simulink model "MuscleEnergyTestModel"  (R2019b)
settings: Solver=ode15s  StartTime=0.0  StopTime=0.005  MaxStep=0.01  RelTol=1e-4  AbsTol=1e-6
values from neighbouring files (symbols this model uses):
  Ahill = 0.25    [MuscleEnergyTest.m]
  c = 0.05    [BodyMechParams.m]
  eref = 0.04    [BodyMechParams.m]
  Fmax = 4000    [MuscleEnergyTest.m]
  FT = 20    [MuscleEnergyTest.m]
  gmax = 1.5    [MuscleEnergyTest.m]
  K = 5    [BodyMechParams.m]
  lopt = 0.055    [MuscleEnergyTest.m]
  lslack = 0.245    [MuscleEnergyTest.m]
  N = 1.5    [BodyMechParams.m]    (also in cmaes.m = size(x,1); mergeCompareEnergyCosts.m = {S.name})
  stim_val = stimulations_val(i)    [MuscleEnergyTest.m]
  v_set = v_simulations(j)    [MuscleEnergyTest.m]
  vmax = 12    [MuscleEnergyTest.m]
  w = 0.56    [BodyMechParams.m]    (also in MuscleEnergyTest.m = 1.039; cmaes.m = ones(size(x,1)))
undefined symbols (not defined in the file or in its folder): iso_short_length
libraries: simulink x1, NeuroMuscularLibrary x1
settings Model: Creator=Nathan  LastModifiedBy=Nathan
settings DataIOCC: SaveFinalState=on  SaveFormat=StructureWithTime  SaveOutput=off  SaveState=on  ReturnWorkspaceOutputs=off

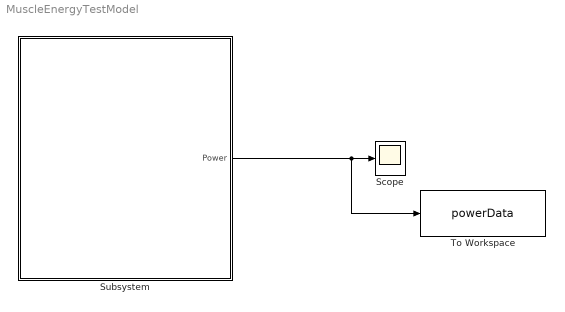
== system MuscleEnergyTestModel ==
  Scope : Scope
  Subsystem : Subsystem  mask{Fmax=Fmax, lopt=lopt, vmax=vmax, lslack=lslack, FT=FT, stim=stim_val, v_set=v_set}
      mask prompts: Fmax "Max Isometric Force in N"; lopt "Optimal Length in m"; vmax "Max Contraction Velocity in m/s"; lslack "Slack Length [m]"; FT "Percent Fast Twitch"; stim "Stimulation value"; v_set "Muscle velocity"
  To Workspace : ToWorkspace  VariableName=powerData  SampleTime=-1
  wires:
  Subsystem/1(Power) -> Scope/1, To Workspace/1

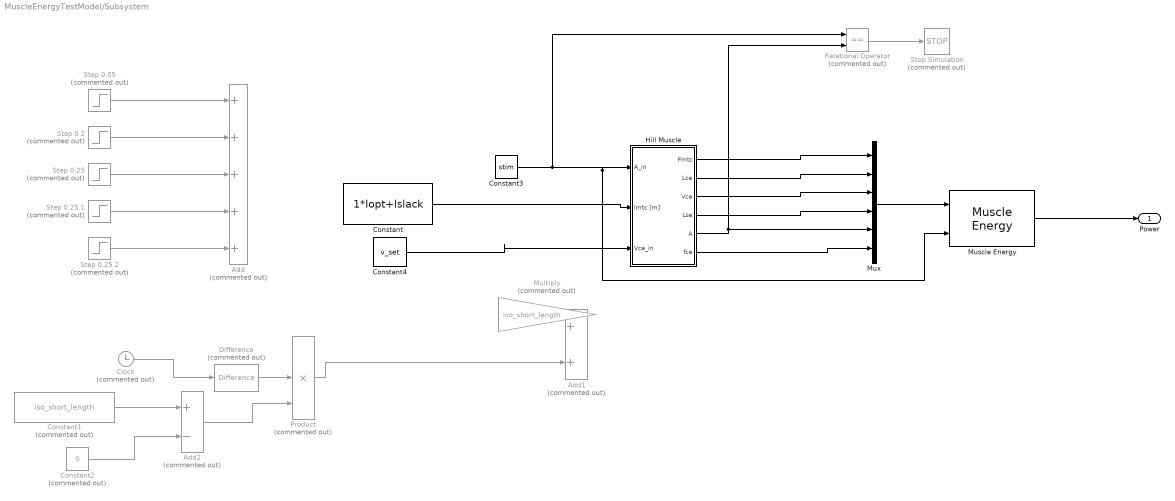
== system MuscleEnergyTestModel/Subsystem ==
  Add : Sum  Commented=on  Inputs=+++++
  Add1 : Sum  Commented=on
  Add2 : Sum  Commented=on  Inputs=+-
  Clock : Clock  Commented=on
      settings: Decimation=10000
  Constant : Constant  Value=1*lopt+lslack
  Constant1 : Constant  Commented=on  Value=iso_short_length
  Constant2 : Constant  Commented=on  Value=0
  Constant3 : Constant  Value=stim
  Constant4 : Constant  Value=v_set
  Difference : simulink/Discrete/Difference  Commented=on  ICPrevInput=0.0  OutMin=[]  OutMax=[]  OutDataType=fixdt(1, 16)  OutScaling=2^-10  DoSatur=off
  Hill Muscle : Subsystem  mask(Hill Type Muscle){Fmax=Fmax, lopt=lopt, vmax=vmax, lslack=lslack}
      mask prompts: Fmax "Max Isometric Force [N]"; lopt "Optimal Length [m]"; vmax "Max Contraction Velocity [m/s]"; lslack "Slack Length [m]"
      mask help:
      | Hill Type Muscle Model. This dialog allows you to specify several muscle-specific parameters. The block also requires several parameters to be defined globally in the matlab workspace:
      |
      | Excitation-contraction coupling parameters:
      | preA: preactivation
      | tau:  delay time constant [s]
      |
      | Contractile element (CE) force-length relationship:
      | w: width [lopt]
      | c: remaining force at +/- width
      |
      | CE force-velocity parameters:
      | N: eccentric force enhancement [Fmax]
      | K: shape factor
      |
      | Series elastic element (SE) force-length relationship
      | eref: tendon reference strain [lslack]
  Multiply : Gain  Commented=on  Gain=iso_short_length
  Muscle Energy : NeuroMuscularLibrary/Muscle Energy  lopt=lopt  FT=FT  Fmax=Fmax  vmax=vmax
  Mux : Mux  Inputs=6
  Product : Product  Commented=on  Inputs=3
  Relational Operator : RelationalOperator  Commented=on  Operator===  OutDataTypeStr=boolean  RndMeth=Simplest
  Step 0.05 : Step  Commented=on  After=0.05  SampleTime=0
  Step 0.2 : Step  Commented=on  Time=4  After=0.2  SampleTime=0
  Step 0.25 : Step  Commented=on  Time=7  After=0.25  SampleTime=0
  Step 0.25 1 : Step  Commented=on  Time=10  After=0.25  SampleTime=0
  Step 0.25 2 : Step  Commented=on  Time=13  After=0.25  SampleTime=0
  Stop Simulation : Stop  Commented=on
  Power : Outport
  wires:
  Mux/1 -> Muscle Energy/1
  Constant3/1 -> Relational Operator/1, Hill Muscle/1(A_in), Muscle Energy/2
  Hill Muscle/3(Vce) -> Mux/3
  Hill Muscle/4(Lse) -> Mux/4
  Hill Muscle/6(fce) -> Mux/6
  Hill Muscle/2(Lce) -> Mux/2
  Hill Muscle/1(Fmtc) -> Mux/1
  Constant/1 -> Hill Muscle/2(lmtc [m])
  Clock/1 -> Difference/1
  Difference/1 -> Product/2
  Product/1 -> Add1/2
  Add2/1 -> Product/3
  Constant1/1 -> Add2/1
  Constant2/1 -> Add2/2
  Muscle Energy/1 -> Power/1
  Step 0.05/1 -> Add/1
  Step 0.25 2/1 -> Add/5
  Step 0.25/1 -> Add/3
  Step 0.25 1/1 -> Add/4
  Step 0.2/1 -> Add/2
  Constant4/1 -> Hill Muscle/3(Vce_in)
  Relational Operator/1 -> Stop Simulation/1
  Hill Muscle/5(A) -> Relational Operator/2, Mux/5

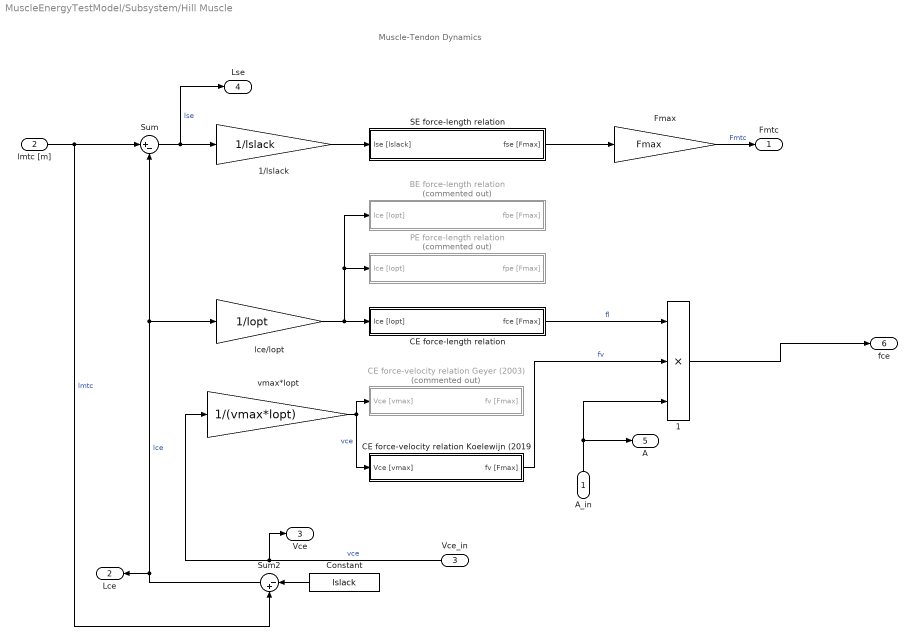
== system MuscleEnergyTestModel/Subsystem/Hill Muscle ==
  note: Muscle-Tendon Dynamics
  A_in : Inport
  lmtc [m] : Inport  Port=2
  Vce_in : Inport  Port=3
  1 : Product  Inputs=***  SaturateOnIntegerOverflow=on  InputSameDT=on  OutDataTypeStr=Inherit: Same as first input
  1/lslack : Gain  Gain=1/lslack  SaturateOnIntegerOverflow=on  OutDataTypeStr=Inherit: Same as input  ParamDataTypeStr=Inherit: Same as input
  BE force-length relation : Subsystem  Commented=on
  CE force-velocity relation Geyer (2003) : Subsystem  Commented=on
  CE force-velocity relation Koelewijn (2019 : Subsystem
  CE force-length relation : Subsystem
  Constant : Constant  Value=lslack
  Fmax : Gain  Gain=Fmax  SaturateOnIntegerOverflow=on  OutDataTypeStr=Inherit: Same as input  ParamDataTypeStr=Inherit: Same as input
  PE force-length relation : Subsystem  Commented=on
  SE force-length relation : Subsystem
  Sum : Sum  Inputs=|+-  SaturateOnIntegerOverflow=on  InputSameDT=on  OutDataTypeStr=Inherit: Same as first input
  Sum2 : Sum  Inputs=|-+  SaturateOnIntegerOverflow=on  InputSameDT=on  OutDataTypeStr=Inherit: Same as first input
  lce/lopt : Gain  Gain=1/lopt  SaturateOnIntegerOverflow=on  OutDataTypeStr=Inherit: Same as input  ParamDataTypeStr=Inherit: Same as input
  vmax*lopt : Gain  Gain=1/(vmax*lopt)  SaturateOnIntegerOverflow=on  OutDataTypeStr=Inherit: Same as input  ParamDataTypeStr=Inherit: Same as input
  Fmtc : Outport  InitialOutput=0
  Lce : Outport  Port=2  InitialOutput=0
  Vce : Outport  Port=3  InitialOutput=0
  Lse : Outport  Port=4  InitialOutput=0
  A : Outport  Port=5  InitialOutput=0
  fce : Outport  Port=6
  wires:
  Sum2/1 -> Sum/2, lce/lopt/1, Lce/1  "lce"
  Sum/1 -> 1/lslack/1, Lse/1  "lse"
  lce/lopt/1 -> CE force-length relation/1(lce [lopt]), BE force-length relation/1(lce [lopt]), PE force-length relation/1(lce [lopt])
  Vce_in/1 -> vmax*lopt/1, Vce/1  "vce"
  lmtc [m]/1 -> Sum2/2, Sum/1  "lmtc"
  Fmax/1 -> Fmtc/1  "Fmtc"
  1/lslack/1 -> SE force-length relation/1(lse [lslack])
  SE force-length relation/1(fse [Fmax]) -> Fmax/1
  Constant/1 -> Sum2/1
  CE force-length relation/1(fce [Fmax]) -> 1/1  "fl"
  1/1 -> fce/1
  A_in/1 -> 1/3, A/1
  vmax*lopt/1 -> CE force-velocity relation Koelewijn (2019/1(Vce [vmax]), CE force-velocity relation Geyer (2003)/1(Vce [vmax])  "vce"
  CE force-velocity relation Koelewijn (2019/1(fv [Fmax]) -> 1/2  "fv"

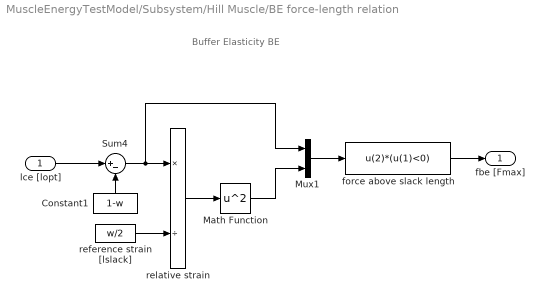
== system MuscleEnergyTestModel/Subsystem/Hill Muscle/BE force-length relation ==
  note: Buffer Elasticity BE
  lce [lopt] : Inport
  Constant1 : Constant  Value=1-w
  Math Function : Math  Operator=square  SaturateOnIntegerOverflow=on
  Mux1 : Mux  Inputs=2
  Sum4 : Sum  Inputs=|+-  SaturateOnIntegerOverflow=on  InputSameDT=on  OutDataTypeStr=Inherit: Same as first input
  force above slack length : Fcn  Expr=u(2)*(u(1)<0)
  reference strain [lslack] : Constant  Value=w/2
  relative strain : Product  Inputs=*/
  fbe [Fmax] : Outport
  wires:
  lce [lopt]/1 -> Sum4/1
  Mux1/1 -> force above slack length/1
  force above slack length/1 -> fbe [Fmax]/1
  Math Function/1 -> Mux1/2
  relative strain/1 -> Math Function/1
  reference strain [lslack]/1 -> relative strain/2
  Sum4/1 -> relative strain/1, Mux1/1
  Constant1/1 -> Sum4/2

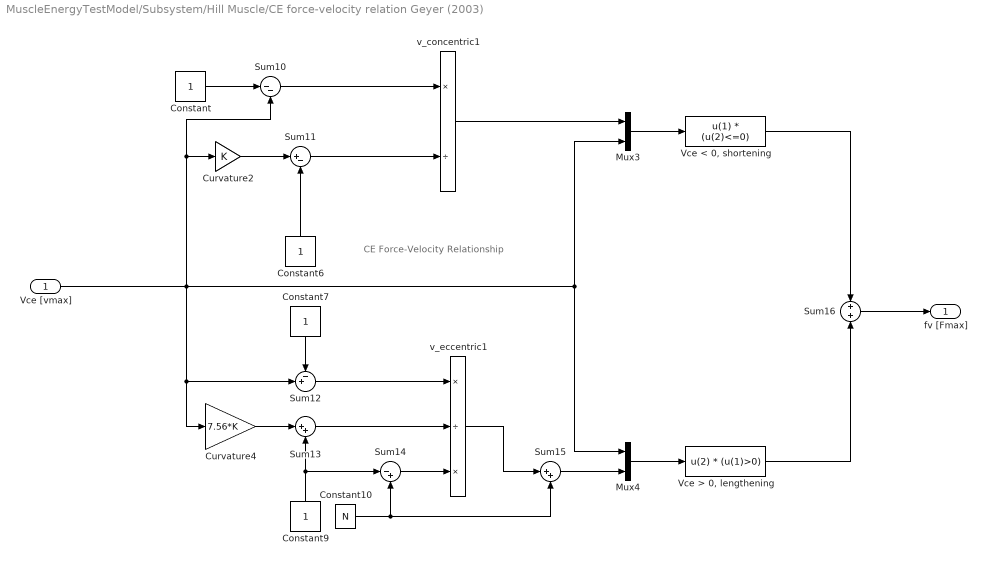
== system MuscleEnergyTestModel/Subsystem/Hill Muscle/CE force-velocity relation Geyer (2003) ==
  note: CE Force-Velocity Relationship
  Vce [vmax] : Inport
  Constant{,6..7,9} (4 alike) : Constant
  Constant10 : Constant  Value=N
  Curvature2 : Gain  Gain=K  SaturateOnIntegerOverflow=on  OutDataTypeStr=Inherit: Same as input  ParamDataTypeStr=Inherit: Same as input
  Curvature4 : Gain  Gain=7.56*K  SaturateOnIntegerOverflow=on  OutDataTypeStr=Inherit: Same as input  ParamDataTypeStr=Inherit: Same as input
  Mux3 : Mux  Inputs=2
  Mux4 : Mux  Inputs=2
  Sum10 : Sum  Inputs=|--  SaturateOnIntegerOverflow=on  InputSameDT=on  OutDataTypeStr=Inherit: Same as first input
  Sum11 : Sum  Inputs=|+-  SaturateOnIntegerOverflow=on  InputSameDT=on  OutDataTypeStr=Inherit: Same as first input
  Sum12 : Sum  Inputs=-+|  SaturateOnIntegerOverflow=on  InputSameDT=on  OutDataTypeStr=Inherit: Same as first input
  Sum13 : Sum  Inputs=|++  SaturateOnIntegerOverflow=on  InputSameDT=on  OutDataTypeStr=Inherit: Same as first input
  Sum14 : Sum  Inputs=|-+  SaturateOnIntegerOverflow=on  InputSameDT=on  OutDataTypeStr=Inherit: Same as first input
  Sum15 : Sum  Inputs=|++  SaturateOnIntegerOverflow=on  InputSameDT=on  OutDataTypeStr=Inherit: Same as first input
  Sum16 : Sum  SaturateOnIntegerOverflow=on  InputSameDT=on  OutDataTypeStr=Inherit: Same as first input
  "Vce < 0, shortening" : Fcn  Expr=u(1) * (u(2)<=0)
  "Vce > 0, lengthening" : Fcn  Expr=u(2) * (u(1)>0)
  v_concentric1 : Product  Inputs=*/
  v_eccentric1 : Product  Inputs=*/*
  fv [Fmax] : Outport
  wires:
  Constant/1 -> Sum10/1
  Sum10/1 -> v_concentric1/1
  Curvature2/1 -> Sum11/1
  Constant6/1 -> Sum11/2
  Sum11/1 -> v_concentric1/2
  Mux3/1 -> "Vce < 0, shortening"/1
  v_concentric1/1 -> Mux3/1
  Curvature4/1 -> Sum13/1
  Sum12/1 -> v_eccentric1/1
  Constant9/1 -> Sum14/1, Sum13/2
  Vce [vmax]/1 -> Curvature4/1, Sum12/2, Sum10/2, Curvature2/1, Mux3/2, Mux4/1
  Sum13/1 -> v_eccentric1/2
  Mux4/1 -> "Vce > 0, lengthening"/1
  Constant7/1 -> Sum12/1
  v_eccentric1/1 -> Sum15/1
  Constant10/1 -> Sum15/2, Sum14/2
  Sum14/1 -> v_eccentric1/3
  Sum15/1 -> Mux4/2
  "Vce < 0, shortening"/1 -> Sum16/1
  "Vce > 0, lengthening"/1 -> Sum16/2
  Sum16/1 -> fv [Fmax]/1

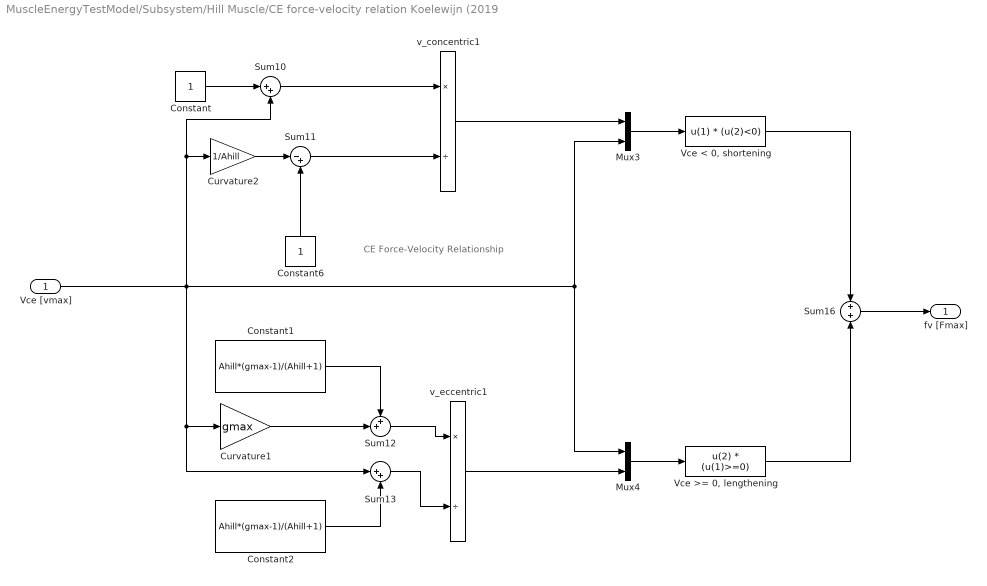
== system MuscleEnergyTestModel/Subsystem/Hill Muscle/CE force-velocity relation Koelewijn (2019 ==
  note: CE Force-Velocity Relationship
  Vce [vmax] : Inport
  Constant : Constant
  Constant1 : Constant  Value=Ahill*(gmax-1)/(Ahill+1)
  Constant2 : Constant  Value=Ahill*(gmax-1)/(Ahill+1)
  Constant6 : Constant
  Curvature1 : Gain  Gain=gmax  SaturateOnIntegerOverflow=on  OutDataTypeStr=Inherit: Same as input  ParamDataTypeStr=Inherit: Same as input
  Curvature2 : Gain  Gain=1/Ahill  SaturateOnIntegerOverflow=on  OutDataTypeStr=Inherit: Same as input  ParamDataTypeStr=Inherit: Same as input
  Mux3 : Mux  Inputs=2
  Mux4 : Mux  Inputs=2
  Sum10 : Sum  Inputs=|++  SaturateOnIntegerOverflow=on  InputSameDT=on  OutDataTypeStr=Inherit: Same as first input
  Sum11 : Sum  Inputs=|-+  SaturateOnIntegerOverflow=on  InputSameDT=on  OutDataTypeStr=Inherit: Same as first input
  Sum12 : Sum  Inputs=++|  SaturateOnIntegerOverflow=on  InputSameDT=on  OutDataTypeStr=Inherit: Same as first input
  Sum13 : Sum  Inputs=|++  SaturateOnIntegerOverflow=on  InputSameDT=on  OutDataTypeStr=Inherit: Same as first input
  Sum16 : Sum  SaturateOnIntegerOverflow=on  InputSameDT=on  OutDataTypeStr=Inherit: Same as first input
  "Vce < 0, shortening" : Fcn  Expr=u(1) * (u(2)<0)
  "Vce >= 0, lengthening" : Fcn  Expr=u(2) * (u(1)>=0)
  v_concentric1 : Product  Inputs=*/
  v_eccentric1 : Product  Inputs=*/
  fv [Fmax] : Outport
  wires:
  Sum16/1 -> fv [Fmax]/1
  "Vce >= 0, lengthening"/1 -> Sum16/2
  "Vce < 0, shortening"/1 -> Sum16/1
  v_eccentric1/1 -> Mux4/2
  Constant1/1 -> Sum12/1
  Mux4/1 -> "Vce >= 0, lengthening"/1
  Sum13/1 -> v_eccentric1/2
  Constant2/1 -> Sum13/2
  Sum12/1 -> v_eccentric1/1
  Vce [vmax]/1 -> Mux4/1, Mux3/2, Sum10/2, Curvature2/1, Sum13/1, Curvature1/1
  v_concentric1/1 -> Mux3/1
  Mux3/1 -> "Vce < 0, shortening"/1
  Sum11/1 -> v_concentric1/2
  Constant6/1 -> Sum11/2
  Curvature2/1 -> Sum11/1
  Sum10/1 -> v_concentric1/1
  Constant/1 -> Sum10/1
  Curvature1/1 -> Sum12/2

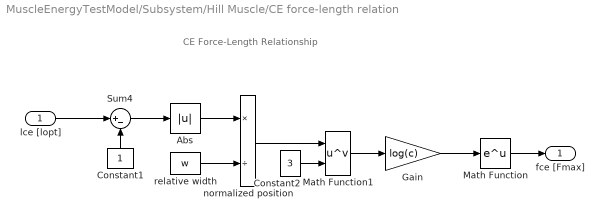
== system MuscleEnergyTestModel/Subsystem/Hill Muscle/CE force-length relation ==
  note: CE Force-Length Relationship
  lce [lopt] : Inport
  Abs : Abs
  Constant1 : Constant
  Constant2 : Constant  Value=3
  Gain : Gain  Gain=log(c)
  Math Function : Math  SaturateOnIntegerOverflow=on
  Math Function1 : Math  Operator=pow  SaturateOnIntegerOverflow=on
  Sum4 : Sum  Inputs=|+-  SaturateOnIntegerOverflow=on  InputSameDT=on  OutDataTypeStr=Inherit: Same as first input
  normalized position : Product  Inputs=*/
  relative width : Constant  Value=w
  fce [Fmax] : Outport
  wires:
  lce [lopt]/1 -> Sum4/1
  relative width/1 -> normalized position/2
  Constant1/1 -> Sum4/2
  Sum4/1 -> Abs/1
  Abs/1 -> normalized position/1
  normalized position/1 -> Math Function1/1
  Constant2/1 -> Math Function1/2
  Math Function1/1 -> Gain/1
  Gain/1 -> Math Function/1
  Math Function/1 -> fce [Fmax]/1

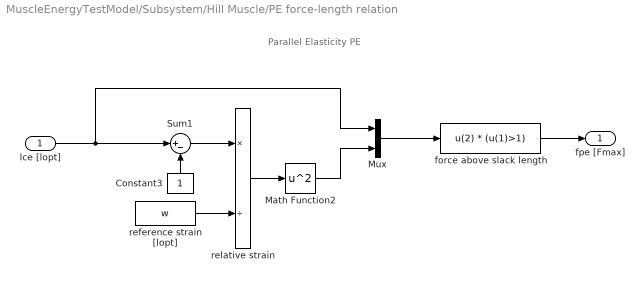
== system MuscleEnergyTestModel/Subsystem/Hill Muscle/PE force-length relation ==
  note: Parallel Elasticity PE
  lce [lopt] : Inport
  Constant3 : Constant
  Math Function2 : Math  Operator=square  SaturateOnIntegerOverflow=on
  Mux : Mux  Inputs=2
  Sum1 : Sum  Inputs=|+-  SaturateOnIntegerOverflow=on  InputSameDT=on  OutDataTypeStr=Inherit: Same as first input
  force above slack length : Fcn  Expr=u(2) * (u(1)>1)
  reference strain [lopt] : Constant  Value=w
  relative strain : Product  Inputs=*/
  fpe [Fmax] : Outport
  wires:
  Mux/1 -> force above slack length/1
  lce [lopt]/1 -> Mux/1, Sum1/1
  Constant3/1 -> Sum1/2
  Sum1/1 -> relative strain/1
  reference strain [lopt]/1 -> relative strain/2
  relative strain/1 -> Math Function2/1
  Math Function2/1 -> Mux/2
  force above slack length/1 -> fpe [Fmax]/1

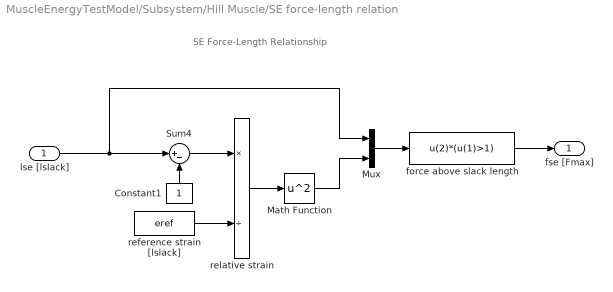
== system MuscleEnergyTestModel/Subsystem/Hill Muscle/SE force-length relation ==
  note: SE Force-Length Relationship
  lse [lslack] : Inport
  Constant1 : Constant
  Math Function : Math  Operator=square  SaturateOnIntegerOverflow=on
  Mux : Mux  Inputs=2
  Sum4 : Sum  Inputs=|+-  SaturateOnIntegerOverflow=on  InputSameDT=on  OutDataTypeStr=Inherit: Same as first input
  force above slack length : Fcn  Expr=u(2)*(u(1)>1)
  reference strain [lslack] : Constant  Value=eref
  relative strain : Product  Inputs=*/
  fse [Fmax] : Outport
  wires:
  Mux/1 -> force above slack length/1
  force above slack length/1 -> fse [Fmax]/1
  Math Function/1 -> Mux/2
  lse [lslack]/1 -> Mux/1, Sum4/1
  relative strain/1 -> Math Function/1
  reference strain [lslack]/1 -> relative strain/2
  Sum4/1 -> relative strain/1
  Constant1/1 -> Sum4/2
